simulink library "simetranss"  (R2024b)
settings: Solver=VariableStepAuto  StartTime=0.0  StopTime=10.0  RelTol=1e-3
PostLoadFcn:
  | Ts=1e-6
InitFcn:
  | Ts=1e-6
undefined symbols (not defined in the file): C, C_601, C_603, C_606, CC, Csnu, Csnubber, DiscIntNeverNeededParam, DPL, DPL1ph, FluxTable, ft2km, gcbh, h, Half, Imap2, L, L_601, L_603, L_606, Lbase, LpejoSw, Newton, R_601, R_603, R_606, Raphson, ResistanceM, Roff, Ron, RotorAngles, Rsnu, Rsnubber, Rt4, SampleTime, simetran, sps, sps_rtmsupport, StatorCurrents, T_2wind_ratio, T_Lpu, T_Lpu_pri, T_Rpu, T_Rpu_pri, T_Vpri, T_Vpri_15comp, T_Vsec, Ti, Ts_Power, Z, Zbase, Zm
libraries: fl_lib x248, ee_lib x146, nesl_utility x122, $bdroot x29, simulink x15, eeGeneralControl x2, spsStairGeneratorLib x2, artemis x1
(part 7 of 12)

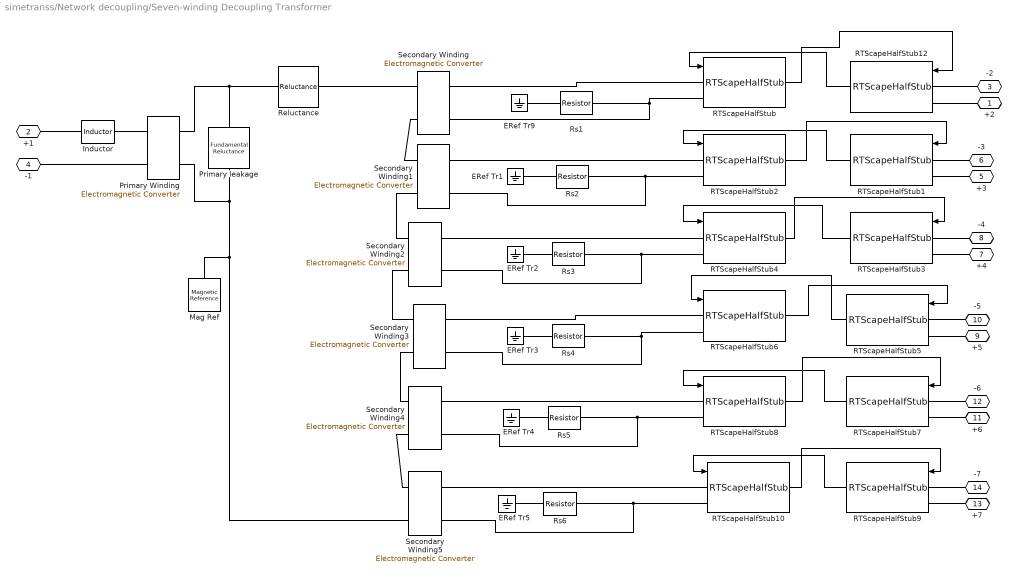
== system simetranss/Network decoupling/Seven-winding Decoupling Transformer ==
  ERef Tr{1..5,9} (6 alike) : fl_lib/Electrical/Electrical Elements/Electrical Reference
  Inductor : fl_lib/Electrical/Electrical Elements/Inductor  l=RLpri(2) H  r=RLpri(1) Ohm  g=1e-9 1/Ohm  i_specify=off  i_priority=None  i=0 A  i_nominal_specify=off  i_nominal_value=1  i_nominal_unit=A  v_specify=off  v_priority=None  v=0 V  v_nominal_specify=off  v_nominal_value=1  v_nominal_unit=V  i_L_specify=off  i_L_priority=High  i_L=0 A  i_L_nominal_specify=off  i_L_nominal_value=1  i_L_nominal_unit=A
  Mag Ref : fl_lib/Magnetic/Magnetic Elements/Magnetic Reference
      settings: InternalSimscapePortConfiguration="{\"Bottom\":[],\"Left\":[{\"id\":\"M\",\"label\":\"\",\"type\":\"foundation.magnetic.magnetic\"}],\"Right\":[],\"Top\":[]}"
  Primary Winding : fl_lib/Magnetic/Magnetic Elements/Electromagnetic Converter  Nw=Vwdn(1)  i_specify=off  i_priority=High  i=0 A  i_nominal_specify=off  i_nominal_value=1  i_nominal_unit=A  v_specify=off  v_priority=High  v=0 V  v_nominal_specify=off  v_nominal_value=1  v_nominal_unit=V  mmf_specify=off  mmf_priority=High  mmf=0 A  mmf_nominal_specify=off  mmf_nominal_value=1  mmf_nominal_unit=A  phi_specify=off  phi_priority=High  phi=0 Wb  phi_nominal_specify=off  phi_nominal_value=1  phi_nominal_unit=Wb
      settings: InternalSimscapePortConfiguration="{\"Bottom\":[],\"Left\":[{\"id\":\"p\",\"label\":\"+\",\"type\":\"foundation.electrical.electrical\"},{\"id\":\"n\",\"label\":\"-\",\"type\":\"foundation.electrical.electrical\"}],\"Right\":[{\"id\":\"N\",\"label\":\"N\",\"type\":\"foundation.magnetic.magnetic\"},{\"id\":\"S\",\"label\":\"S\",\"type\":\"foundation.magnetic.magnetic\"}],\"Top\":[]}"
  Primary leakage : fl_lib/Magnetic/Magnetic Elements/Fundamental Reluctance  R=1e8 1/H  phi_specify=off  phi_priority=None  phi=0 Wb  phi_nominal_specify=off  phi_nominal_value=1  phi_nominal_unit=Wb  mmf_specify=off  mmf_priority=None  mmf=0 A  mmf_nominal_specify=off  mmf_nominal_value=1  mmf_nominal_unit=A
      settings: InternalSimscapePortConfiguration="{\"Bottom\":[],\"Left\":[{\"id\":\"N\",\"label\":\"N\",\"type\":\"foundation.magnetic.magnetic\"}],\"Right\":[{\"id\":\"S\",\"label\":\"S\",\"type\":\"foundation.magnetic.magnetic\"}],\"Top\":[]}"
  RTScapeHalfStub : $bdroot/Network decoupling/RTScapeHalfStub  Phases=2 with differential inputs  pu=off  L=Lwdn(1)  Lpu=0.03  R=Rwdn(1)  Rpu=0.02  S_base=1e5  V_base=1000  F_base=60  Ts=Ts
  RTScapeHalfStub1 : $bdroot/Network decoupling/RTScapeHalfStub  Phases=2 with differential inputs  pu=off  L=Lwdn(2)  Lpu=0.03  R=Rwdn(2)  Rpu=0.02  S_base=1e5  V_base=1000  F_base=60  Ts=Ts
  RTScapeHalfStub10 : $bdroot/Network decoupling/RTScapeHalfStub  Phases=2 with differential inputs  pu=off  L=Lwdn(6)  Lpu=0.03  R=Rwdn(6)  Rpu=0.02  S_base=1e5  V_base=1000  F_base=60  Ts=Ts
  RTScapeHalfStub12 : $bdroot/Network decoupling/RTScapeHalfStub  Phases=2 with differential inputs  pu=off  L=Lwdn(1)  Lpu=0.03  R=Rwdn(1)  Rpu=0.02  S_base=1e5  V_base=1000  F_base=60  Ts=Ts
  RTScapeHalfStub2 : $bdroot/Network decoupling/RTScapeHalfStub  Phases=2 with differential inputs  pu=off  L=Lwdn(2)  Lpu=0.03  R=Rwdn(2)  Rpu=0.02  S_base=1e5  V_base=1000  F_base=60  Ts=Ts
  RTScapeHalfStub3 : $bdroot/Network decoupling/RTScapeHalfStub  Phases=2 with differential inputs  pu=off  L=Lwdn(3)  Lpu=0.03  R=Rwdn(3)  Rpu=0.02  S_base=1e5  V_base=1000  F_base=60  Ts=Ts
  RTScapeHalfStub4 : $bdroot/Network decoupling/RTScapeHalfStub  Phases=2 with differential inputs  pu=off  L=Lwdn(3)  Lpu=0.03  R=Rwdn(3)  Rpu=0.02  S_base=1e5  V_base=1000  F_base=60  Ts=Ts
  RTScapeHalfStub5 : $bdroot/Network decoupling/RTScapeHalfStub  Phases=2 with differential inputs  pu=off  L=Lwdn(4)  Lpu=0.03  R=Rwdn(4)  Rpu=0.02  S_base=1e5  V_base=1000  F_base=60  Ts=Ts
  RTScapeHalfStub6 : $bdroot/Network decoupling/RTScapeHalfStub  Phases=2 with differential inputs  pu=off  L=Lwdn(4)  Lpu=0.03  R=Rwdn(4)  Rpu=0.02  S_base=1e5  V_base=1000  F_base=60  Ts=Ts
  RTScapeHalfStub7 : $bdroot/Network decoupling/RTScapeHalfStub  Phases=2 with differential inputs  pu=off  L=Lwdn(5)  Lpu=0.03  R=Rwdn(5)  Rpu=0.02  S_base=1e5  V_base=1000  F_base=60  Ts=Ts
  RTScapeHalfStub8 : $bdroot/Network decoupling/RTScapeHalfStub  Phases=2 with differential inputs  pu=off  L=Lwdn(5)  Lpu=0.03  R=Rwdn(5)  Rpu=0.02  S_base=1e5  V_base=1000  F_base=60  Ts=Ts
  RTScapeHalfStub9 : $bdroot/Network decoupling/RTScapeHalfStub  Phases=2 with differential inputs  pu=off  L=Lwdn(6)  Lpu=0.03  R=Rwdn(6)  Rpu=0.02  S_base=1e5  V_base=1000  F_base=60  Ts=Ts
  Reluctance : fl_lib/Magnetic/Magnetic Elements/Reluctance  g=0.2 m  CSA=0.035*0.035 m^2  mur=8000  phi_specify=off  phi_priority=High  phi=0 Wb  phi_nominal_specify=off  phi_nominal_value=1  phi_nominal_unit=Wb  mmf_specify=off  mmf_priority=High  mmf=0 A  mmf_nominal_specify=off  mmf_nominal_value=1  mmf_nominal_unit=A
      settings: InternalSimscapePortConfiguration="{\"Bottom\":[],\"Left\":[{\"id\":\"N\",\"label\":\"N\",\"type\":\"foundation.magnetic.magnetic\"}],\"Right\":[{\"id\":\"S\",\"label\":\"S\",\"type\":\"foundation.magnetic.magnetic\"}],\"Top\":[]}"
  Rs{1..6} (6 alike) : fl_lib/Electrical/Electrical Elements/Resistor  R=Rearth Ohm  i_specify=off  i_priority=High  i=0 A  i_nominal_specify=off  i_nominal_value=1  i_nominal_unit=A  v_specify=off  v_priority=High  v=0 V  v_nominal_specify=off  v_nominal_value=1  v_nominal_unit=V
  Secondary Winding : fl_lib/Magnetic/Magnetic Elements/Electromagnetic Converter  Nw=Vwdn(1)  i_specify=off  i_priority=High  i=0 A  i_nominal_specify=off  i_nominal_value=1  i_nominal_unit=A  v_specify=off  v_priority=High  v=0 V  v_nominal_specify=off  v_nominal_value=1  v_nominal_unit=V  mmf_specify=off  mmf_priority=High  mmf=0 A  mmf_nominal_specify=off  mmf_nominal_value=1  mmf_nominal_unit=A  phi_specify=off  phi_priority=High  phi=0 Wb  phi_nominal_specify=off  phi_nominal_value=1  phi_nominal_unit=Wb
      settings: InternalSimscapePortConfiguration="{\"Bottom\":[],\"Left\":[{\"id\":\"p\",\"label\":\"+\",\"type\":\"foundation.electrical.electrical\"},{\"id\":\"n\",\"label\":\"-\",\"type\":\"foundation.electrical.electrical\"}],\"Right\":[{\"id\":\"N\",\"label\":\"N\",\"type\":\"foundation.magnetic.magnetic\"},{\"id\":\"S\",\"label\":\"S\",\"type\":\"foundation.magnetic.magnetic\"}],\"Top\":[]}"
  Secondary Winding1 : fl_lib/Magnetic/Magnetic Elements/Electromagnetic Converter  Nw=Vwdn(2)  i_specify=off  i_priority=High  i=0 A  i_nominal_specify=off  i_nominal_value=1  i_nominal_unit=A  v_specify=off  v_priority=High  v=0 V  v_nominal_specify=off  v_nominal_value=1  v_nominal_unit=V  mmf_specify=off  mmf_priority=High  mmf=0 A  mmf_nominal_specify=off  mmf_nominal_value=1  mmf_nominal_unit=A  phi_specify=off  phi_priority=High  phi=0 Wb  phi_nominal_specify=off  phi_nominal_value=1  phi_nominal_unit=Wb
      settings: InternalSimscapePortConfiguration="{\"Bottom\":[],\"Left\":[{\"id\":\"p\",\"label\":\"+\",\"type\":\"foundation.electrical.electrical\"},{\"id\":\"n\",\"label\":\"-\",\"type\":\"foundation.electrical.electrical\"}],\"Right\":[{\"id\":\"N\",\"label\":\"N\",\"type\":\"foundation.magnetic.magnetic\"},{\"id\":\"S\",\"label\":\"S\",\"type\":\"foundation.magnetic.magnetic\"}],\"Top\":[]}"
  Secondary Winding2 : fl_lib/Magnetic/Magnetic Elements/Electromagnetic Converter  Nw=Vwdn(3)  i_specify=off  i_priority=High  i=0 A  i_nominal_specify=off  i_nominal_value=1  i_nominal_unit=A  v_specify=off  v_priority=High  v=0 V  v_nominal_specify=off  v_nominal_value=1  v_nominal_unit=V  mmf_specify=off  mmf_priority=High  mmf=0 A  mmf_nominal_specify=off  mmf_nominal_value=1  mmf_nominal_unit=A  phi_specify=off  phi_priority=High  phi=0 Wb  phi_nominal_specify=off  phi_nominal_value=1  phi_nominal_unit=Wb
      settings: InternalSimscapePortConfiguration="{\"Bottom\":[],\"Left\":[{\"id\":\"p\",\"label\":\"+\",\"type\":\"foundation.electrical.electrical\"},{\"id\":\"n\",\"label\":\"-\",\"type\":\"foundation.electrical.electrical\"}],\"Right\":[{\"id\":\"N\",\"label\":\"N\",\"type\":\"foundation.magnetic.magnetic\"},{\"id\":\"S\",\"label\":\"S\",\"type\":\"foundation.magnetic.magnetic\"}],\"Top\":[]}"
  Secondary Winding3 : fl_lib/Magnetic/Magnetic Elements/Electromagnetic Converter  Nw=Vwdn(4)  i_specify=off  i_priority=High  i=0 A  i_nominal_specify=off  i_nominal_value=1  i_nominal_unit=A  v_specify=off  v_priority=High  v=0 V  v_nominal_specify=off  v_nominal_value=1  v_nominal_unit=V  mmf_specify=off  mmf_priority=High  mmf=0 A  mmf_nominal_specify=off  mmf_nominal_value=1  mmf_nominal_unit=A  phi_specify=off  phi_priority=High  phi=0 Wb  phi_nominal_specify=off  phi_nominal_value=1  phi_nominal_unit=Wb
      settings: InternalSimscapePortConfiguration="{\"Bottom\":[],\"Left\":[{\"id\":\"p\",\"label\":\"+\",\"type\":\"foundation.electrical.electrical\"},{\"id\":\"n\",\"label\":\"-\",\"type\":\"foundation.electrical.electrical\"}],\"Right\":[{\"id\":\"N\",\"label\":\"N\",\"type\":\"foundation.magnetic.magnetic\"},{\"id\":\"S\",\"label\":\"S\",\"type\":\"foundation.magnetic.magnetic\"}],\"Top\":[]}"
  Secondary Winding4 : fl_lib/Magnetic/Magnetic Elements/Electromagnetic Converter  Nw=Vwdn(5)  i_specify=off  i_priority=High  i=0 A  i_nominal_specify=off  i_nominal_value=1  i_nominal_unit=A  v_specify=off  v_priority=High  v=0 V  v_nominal_specify=off  v_nominal_value=1  v_nominal_unit=V  mmf_specify=off  mmf_priority=High  mmf=0 A  mmf_nominal_specify=off  mmf_nominal_value=1  mmf_nominal_unit=A  phi_specify=off  phi_priority=High  phi=0 Wb  phi_nominal_specify=off  phi_nominal_value=1  phi_nominal_unit=Wb
      settings: InternalSimscapePortConfiguration="{\"Bottom\":[],\"Left\":[{\"id\":\"p\",\"label\":\"+\",\"type\":\"foundation.electrical.electrical\"},{\"id\":\"n\",\"label\":\"-\",\"type\":\"foundation.electrical.electrical\"}],\"Right\":[{\"id\":\"N\",\"label\":\"N\",\"type\":\"foundation.magnetic.magnetic\"},{\"id\":\"S\",\"label\":\"S\",\"type\":\"foundation.magnetic.magnetic\"}],\"Top\":[]}"
  Secondary Winding5 : fl_lib/Magnetic/Magnetic Elements/Electromagnetic Converter  Nw=Vwdn(6)  i_specify=off  i_priority=High  i=0 A  i_nominal_specify=off  i_nominal_value=1  i_nominal_unit=A  v_specify=off  v_priority=High  v=0 V  v_nominal_specify=off  v_nominal_value=1  v_nominal_unit=V  mmf_specify=off  mmf_priority=High  mmf=0 A  mmf_nominal_specify=off  mmf_nominal_value=1  mmf_nominal_unit=A  phi_specify=off  phi_priority=High  phi=0 Wb  phi_nominal_specify=off  phi_nominal_value=1  phi_nominal_unit=Wb
      settings: InternalSimscapePortConfiguration="{\"Bottom\":[],\"Left\":[{\"id\":\"p\",\"label\":\"+\",\"type\":\"foundation.electrical.electrical\"},{\"id\":\"n\",\"label\":\"-\",\"type\":\"foundation.electrical.electrical\"}],\"Right\":[{\"id\":\"N\",\"label\":\"N\",\"type\":\"foundation.magnetic.magnetic\"},{\"id\":\"S\",\"label\":\"S\",\"type\":\"foundation.magnetic.magnetic\"}],\"Top\":[]}"
  +2 : PMIOPort  Side=Right
  +1 : PMIOPort  Port=2  Side=Left
  -2 : PMIOPort  Port=3  Side=Right
  -1 : PMIOPort  Port=4  Side=Left
  +3 : PMIOPort  Port=5  Side=Right
  -3 : PMIOPort  Port=6  Side=Right
  +4 : PMIOPort  Port=7  Side=Right
  -4 : PMIOPort  Port=8  Side=Right
  +5 : PMIOPort  Port=9  Side=Right
  -5 : PMIOPort  Port=10  Side=Right
  +6 : PMIOPort  Port=11  Side=Right
  -6 : PMIOPort  Port=12  Side=Right
  +7 : PMIOPort  Port=13  Side=Right
  -7 : PMIOPort  Port=14  Side=Right
  wires:
  RTScapeHalfStub/1 -> RTScapeHalfStub12/1
  RTScapeHalfStub12/1 -> RTScapeHalfStub/1
  RTScapeHalfStub1/1 -> RTScapeHalfStub2/1
  RTScapeHalfStub2/1 -> RTScapeHalfStub1/1
  RTScapeHalfStub4/1 -> RTScapeHalfStub3/1
  RTScapeHalfStub3/1 -> RTScapeHalfStub4/1
  RTScapeHalfStub5/1 -> RTScapeHalfStub6/1
  RTScapeHalfStub6/1 -> RTScapeHalfStub5/1
  RTScapeHalfStub8/1 -> RTScapeHalfStub7/1
  RTScapeHalfStub7/1 -> RTScapeHalfStub8/1
  RTScapeHalfStub9/1 -> RTScapeHalfStub10/1
  RTScapeHalfStub10/1 -> RTScapeHalfStub9/1
  connections:
  Secondary Winding4/RConn1 -- Secondary Winding5/RConn2
  Secondary Winding3/RConn1 -- Secondary Winding4/RConn2
  Secondary Winding2/RConn1 -- Secondary Winding3/RConn2
  Secondary Winding1/RConn1 -- Secondary Winding2/RConn2
  Secondary Winding1/RConn2 -- Secondary Winding/RConn1
  Reluctance/RConn1 -- Secondary Winding/RConn2
  Primary leakage/RConn1 -- Primary Winding/RConn2 -- Mag Ref/LConn1 -- Secondary Winding5/RConn1
  Primary leakage/LConn1 -- Reluctance/LConn1 -- Primary Winding/RConn1
  -1/RConn1 -- Primary Winding/LConn2
  Inductor/RConn1 -- Primary Winding/LConn1
  Secondary Winding/LConn1 -- RTScapeHalfStub/LConn2 -- Rs1/RConn1
  Rs1/LConn1 -- ERef Tr9/LConn1
  RTScapeHalfStub12/LConn2 -- +2/RConn1
  RTScapeHalfStub12/LConn1 -- -2/RConn1
  RTScapeHalfStub/LConn1 -- Secondary Winding/LConn2
  Rs2/RConn1 -- RTScapeHalfStub2/LConn2 -- Secondary Winding1/LConn1
  RTScapeHalfStub2/LConn1 -- Secondary Winding1/LConn2
  RTScapeHalfStub1/LConn2 -- +3/RConn1
  RTScapeHalfStub1/LConn1 -- -3/RConn1
  Rs2/LConn1 -- ERef Tr1/LConn1
  Rs3/RConn1 -- RTScapeHalfStub4/LConn2 -- Secondary Winding2/LConn1
  ERef Tr2/LConn1 -- Rs3/LConn1
  RTScapeHalfStub4/LConn1 -- Secondary Winding2/LConn2
  RTScapeHalfStub3/LConn1 -- -4/RConn1
  RTScapeHalfStub3/LConn2 -- +4/RConn1
  Rs4/RConn1 -- RTScapeHalfStub6/LConn2 -- Secondary Winding3/LConn1
  RTScapeHalfStub5/LConn1 -- -5/RConn1
  RTScapeHalfStub6/LConn1 -- Secondary Winding3/LConn2
  ERef Tr3/LConn1 -- Rs4/LConn1
  RTScapeHalfStub5/LConn2 -- +5/RConn1
  Rs5/RConn1 -- RTScapeHalfStub8/LConn2 -- Secondary Winding4/LConn1
  RTScapeHalfStub7/LConn2 -- +6/RConn1
  ERef Tr4/LConn1 -- Rs5/LConn1
  RTScapeHalfStub7/LConn1 -- -6/RConn1
  RTScapeHalfStub8/LConn1 -- Secondary Winding4/LConn2
  Rs6/RConn1 -- RTScapeHalfStub10/LConn2 -- Secondary Winding5/LConn1
  RTScapeHalfStub10/LConn1 -- Secondary Winding5/LConn2
  ERef Tr5/LConn1 -- Rs6/LConn1
  RTScapeHalfStub9/LConn1 -- -7/RConn1
  RTScapeHalfStub9/LConn2 -- +7/RConn1
  +1/RConn1 -- Inductor/LConn1

== system simetranss/Network decoupling/Three-Phase 2-Windings Decoupling Transformer ==
  Signal Specification : SignalSpecification  Dimensions=3
  Signal Specification1 : SignalSpecification  Dimensions=3
  Switch : Switch  Criteria=u2 > Threshold  Threshold=0.5  SaturateOnIntegerOverflow=off  InputSameDT=off
  Switch1 : Switch  Criteria=u2 > Threshold  Threshold=0.5  SaturateOnIntegerOverflow=off  InputSameDT=off
  Terminator : Terminator
  Terminator1 : Terminator
  del{1..4} (4 alike) : UnitDelay  SampleTime=Ts  HasFrameUpgradeWarning=on
  hinpri : Ground
  hinsec : Ground
  houtpri : Terminator
  houtsec : Terminator
  path : Constant
  pri : Subsystem
  sec : Subsystem
  ABC : PMIOPort  Side=Left
  N : PMIOPort  Port=2  Side=Left
  abc : PMIOPort  Port=3  Side=Right
  n : PMIOPort  Port=4  Side=Right
  wires:
  pri/1(Out1) -> Signal Specification1/1, Terminator/1, houtpri/1
  sec/1(Out1) -> Terminator1/1, houtsec/1, Signal Specification/1
  Switch/1 -> pri/1(In1)
  del1/1 -> Switch/3
  hinpri/1 -> del4/1
  path/1 -> Switch/2, Switch1/2
  del2/1 -> Switch1/3
  Switch1/1 -> sec/1(In1)
  hinsec/1 -> del3/1
  Signal Specification/1 -> del1/1
  Signal Specification1/1 -> del2/1
  del3/1 -> Switch1/1
  del4/1 -> Switch/1
  connections:
  ABC/RConn1 -- pri/LConn1
  N/RConn1 -- pri/LConn2
  abc/RConn1 -- sec/RConn1
  n/RConn1 -- sec/RConn2

== system simetranss/Passive/MATE Single-Phase Load ==
  C : Subsystem  Commented=on
  RLseries : Subsystem
  a : PMIOPort  Side=Left
  connections:
  C/LConn1 -- a/RConn1 -- RLseries/LConn1

== system simetranss/Passive/MATE Unbalanced Load ==
  C : Subsystem  Commented=on
  RLseries : Subsystem
  abc : PMIOPort  Side=Left
  connections:
  abc/RConn1 -- C/LConn1 -- RLseries/LConn1

== system simetranss/Passive/MATE Unbalanced LoadDEV1 ==
  C : Subsystem  Commented=on
  CD : Subsystem  Commented=on
  RLseries : Subsystem
  RLseriesD : Subsystem
  abc : PMIOPort  Side=Left
  connections:
  abc/RConn1 -- RLseriesD/LConn1 -- RLseries/LConn1 -- CD/LConn1 -- C/LConn1

== system simetranss/Passive/RLC ==
  note: RLC parallel LC parallel
  note: RLC series LC series
  note: L RLseries RLparallel
  note: C RCseries RCparallel
  C : ee_lib/Passive/Capacitor  Commented=on  cap_option=ee.enum.passive.capacitor.capOption.const  c=Capacitance F  Cvec=[1e-05, 1e-06] F  Vvec=[0, 10] V  CV_table_symmetry=ee.enum.passive.capacitor.tableSymmetry.yes  f_vec=[1, 10] kHz  DFext_vec=[.8, 1.2]  enable_C_tol=ee.enum.toleranceApplication.none  averaging_period=0 s  C_tol=5  tol_distribution=ee.enum.toleranceDistribution.uniform  nSigma=4  r=Resistance2 Ohm  g=0 1/Ohm  enable_operating_limits=ee.enum.enable.no  operating_limit_action=ee.enum.passive.reportOpLim.warn  max_working_voltage_range=[-25, 25] V  power_rating=1 W  maxTemperature=85 degC  thermalEnable=false  thermalMass=1 J/K  fault_action=simscape.enum.assert.action.none  t_fault=1 s  i_specify=off  i_priority=None  i=0 A  i_nominal_specify=off  i_nominal_value=1  i_nominal_unit=A  v_specify=off  v_priority=None  v=0 V  v_nominal_specify=off  v_nominal_value=1  v_nominal_unit=V  vc_specify=off  vc_priority=High  vc=0 V  vc_nominal_specify=off  vc_nominal_value=1  vc_nominal_unit=V  T_specify=off  T_priority=None  T=298.15 K  T_nominal_specify=off  T_nominal_value=1  T_nominal_unit=K
  L : ee_lib/Passive/Inductor  l=Inductance H  enable_L_tol=ee.enum.toleranceApplication.none  L_tol=20  tol_distribution=ee.enum.toleranceDistribution.uniform  nSigma=4  r=Resistance2 Ohm  g=0 1/Ohm  enable_operating_limits=ee.enum.enable.no  operating_limit_action=ee.enum.passive.reportOpLim.warn  max_working_current=1 A  power_rating=1 W  fault_action=simscape.enum.assert.action.none  t_fault=1 s  i_L_specify=off  i_L_priority=High  i_L=0 A  i_L_nominal_specify=off  i_L_nominal_value=1  i_L_nominal_unit=A
  R : ee_lib/Passive/Resistor  R=Resistance Ohm  enable_R_tol=ee.enum.toleranceApplication.none  R_tol=5  tol_distribution=ee.enum.toleranceDistribution.uniform  nSigma=4  enable_operating_limits=ee.enum.enable.no  operating_limit_action=ee.enum.passive.reportOpLim.warn  power_rating=1 W  max_working_voltage=100 V  noise_mode=ee.enum.sources.noise.Disabled  Tdevice=25 degC  sample_time=1e-3 s  repeatability=ee.enum.ic.repeatability.notRepeatable  user_seed=0  auto_seed=3102854422  fault_action=simscape.enum.assert.action.none  t_fault=1 s  power_derating_T1=70 degC  power_derating_T2=155 degC  operating_temperature_range_vec=[-50, 150] degC  alpha=3.93e-3 1/K  Tmeas=25 degC  thermal_mass=100 J/K  temperature_specify=off  temperature_priority=High  temperature=298.15 K  temperature_nominal_specify=off  temperature_nominal_value=1  temperature_nominal_unit=K
  RLCp_1 : ee_lib/Passive/Capacitor  Commented=on  cap_option=ee.enum.passive.capacitor.capOption.const  c=Capacitance F  Cvec=[1e-05, 1e-06] F  Vvec=[0, 10] V  CV_table_symmetry=ee.enum.passive.capacitor.tableSymmetry.yes  f_vec=[1, 10] kHz  DFext_vec=[.8, 1.2]  enable_C_tol=ee.enum.toleranceApplication.none  averaging_period=0 s  C_tol=5  tol_distribution=ee.enum.toleranceDistribution.uniform  nSigma=4  r=0 Ohm  g=1/Resistance2 1/Ohm  enable_operating_limits=ee.enum.enable.no  operating_limit_action=ee.enum.passive.reportOpLim.warn  max_working_voltage_range=[-25, 25] V  power_rating=1 W  maxTemperature=85 degC  thermalEnable=false  thermalMass=1 J/K  fault_action=simscape.enum.assert.action.none  t_fault=1 s  i_specify=off  i_priority=None  i=0 A  i_nominal_specify=off  i_nominal_value=1  i_nominal_unit=A  v_specify=off  v_priority=None  v=0 V  v_nominal_specify=off  v_nominal_value=1  v_nominal_unit=V  vc_specify=off  vc_priority=High  vc=0 V  vc_nominal_specify=off  vc_nominal_value=1  vc_nominal_unit=V  T_specify=off  T_priority=None  T=298.15 K  T_nominal_specify=off  T_nominal_value=1  T_nominal_unit=K
  RLCp_2 : ee_lib/Passive/Inductor  Commented=on  l=Inductance H  enable_L_tol=ee.enum.toleranceApplication.none  L_tol=20  tol_distribution=ee.enum.toleranceDistribution.uniform  nSigma=4  r=0 Ohm  g=0 1/Ohm  enable_operating_limits=ee.enum.enable.no  operating_limit_action=ee.enum.passive.reportOpLim.warn  max_working_current=1 A  power_rating=1 W  fault_action=simscape.enum.assert.action.none  t_fault=1 s  i_L_specify=off  i_L_priority=High  i_L=0 A  i_L_nominal_specify=off  i_L_nominal_value=1  i_L_nominal_unit=A
  RLCs_1 : ee_lib/Passive/Capacitor  Commented=on  cap_option=ee.enum.passive.capacitor.capOption.const  c=Capacitance F  Cvec=[1e-05, 1e-06] F  Vvec=[0, 10] V  CV_table_symmetry=ee.enum.passive.capacitor.tableSymmetry.yes  f_vec=[1, 10] kHz  DFext_vec=[.8, 1.2]  enable_C_tol=ee.enum.toleranceApplication.none  averaging_period=0 s  C_tol=5  tol_distribution=ee.enum.toleranceDistribution.uniform  nSigma=4  r=0 Ohm  g=0 1/Ohm  enable_operating_limits=ee.enum.enable.no  operating_limit_action=ee.enum.passive.reportOpLim.warn  max_working_voltage_range=[-25, 25] V  power_rating=1 W  maxTemperature=85 degC  thermalEnable=false  thermalMass=1 J/K  fault_action=simscape.enum.assert.action.none  t_fault=1 s  i_specify=off  i_priority=None  i=0 A  i_nominal_specify=off  i_nominal_value=1  i_nominal_unit=A  v_specify=off  v_priority=None  v=0 V  v_nominal_specify=off  v_nominal_value=1  v_nominal_unit=V  vc_specify=off  vc_priority=High  vc=0 V  vc_nominal_specify=off  vc_nominal_value=1  vc_nominal_unit=V  T_specify=off  T_priority=None  T=298.15 K  T_nominal_specify=off  T_nominal_value=1  T_nominal_unit=K
  RLCs_2 : ee_lib/Passive/Inductor  Commented=on  l=Inductance H  enable_L_tol=ee.enum.toleranceApplication.none  L_tol=20  tol_distribution=ee.enum.toleranceDistribution.uniform  nSigma=4  r=Resistance2 Ohm  g=0 1/Ohm  enable_operating_limits=ee.enum.enable.no  operating_limit_action=ee.enum.passive.reportOpLim.warn  max_working_current=1 A  power_rating=1 W  fault_action=simscape.enum.assert.action.none  t_fault=1 s  i_L_specify=off  i_L_priority=High  i_L=0 A  i_L_nominal_specify=off  i_L_nominal_value=1  i_L_nominal_unit=A
  + : PMIOPort  Side=Left
  - : PMIOPort  Port=2  Side=Right
  connections:
  C/LConn1 -- +/RConn1 -- R/RConn1 -- L/LConn1 -- RLCs_1/LConn1 -- RLCp_2/LConn1 -- RLCp_1/LConn1
  RLCs_2/LConn1 -- RLCs_1/RConn1
  L/RConn1 -- -/RConn1 -- R/LConn1 -- C/RConn1 -- RLCs_2/RConn1 -- RLCp_2/RConn1 -- RLCp_1/RConn1

== system simetranss/Passive/RLC(3ph) ==
  RLC3 : ee_lib/Passive/RLC Assemblies/RLC (Three-Phase)  port_option=ee.enum.threePhasePort.composite  component_structure=ee.enum.rlc.structure.SeriesRLC  R=Resistance Ohm  L=Inductance H  C=Capacitance F  R_parasitic=0 Ohm  G_parasitic=0 1/Ohm  IL_specify=off  IL_priority=High  IL=[0, 0, 0] A  IL_nominal_specify=off  IL_nominal_value=1  IL_nominal_unit=A  VC_specify=off  VC_priority=High  VC=[0, 0, 0] V  VC_nominal_specify=off  VC_nominal_value=1  VC_nominal_unit=V
      settings: InternalSimscapePortConfiguration="{\"Bottom\":[],\"Left\":[{\"id\":\"N1\",\"label\":\"~1\",\"type\":\"foundation.electrical.three_phase\"}],\"Right\":[{\"id\":\"N2\",\"label\":\"~2\",\"type\":\"foundation.electrical.three_phase\"}],\"Top\":[]}"
  + : PMIOPort  Side=Left
  - : PMIOPort  Port=2  Side=Right
  connections:
  RLC3/RConn1 -- -/RConn1
  RLC3/LConn1 -- +/RConn1

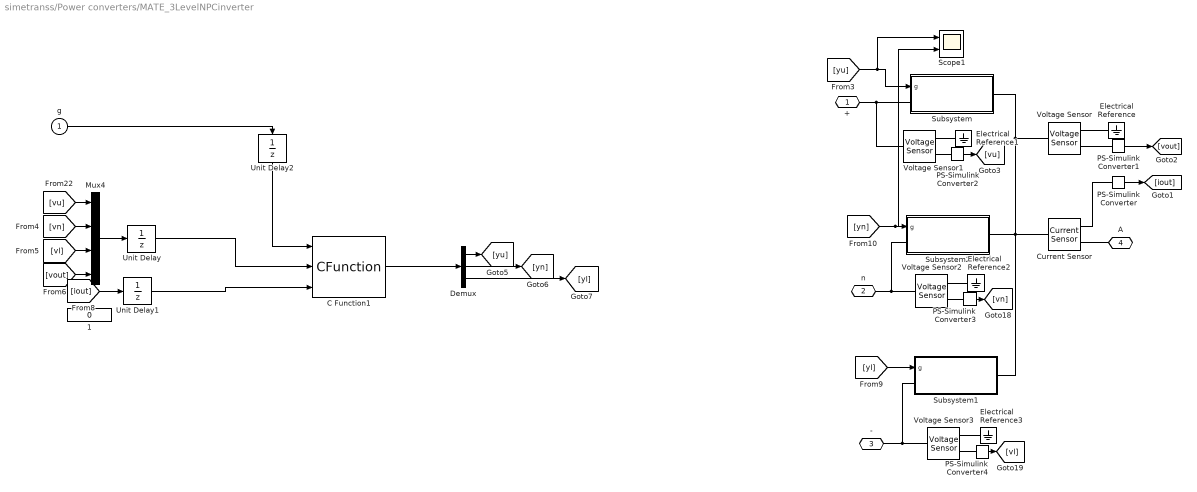
== system simetranss/Power converters/MATE_3LevelNPCinverter ==
  g : Inport
  1 : Constant  Value=0
  C Function1 : CFunction  OutputCode=|  InitializeConditionsCode=status_old=0;  CodegenOutputCode=|  CodegenInitializeConditionsCode=status_old=0;  CustomCodeSettingLocation=ModelConfigurationParameters
      OutputCode=|
      | {
      |     double status;
      | 
      |     //InputRealPtrsType gg      = ssGetInputPortRealSignalPtrs(S,0);
      |     //InputRealPtrsType Vtermm  = ssGetInputPortRealSignalPtrs(S,1);
      |     //InputRealPtrsType ioutt   = ssGetInputPortRealSignalPtrs(S,2);
      |     //InputRealPtrsType tol     = ssGetInputPortRealSignalPtrs(S,3);
      | 
      | 
      |     //real_T            *sw       =  ssGetOutputPortRealSignal(S,0);  // sw
      |     //real_T			  *stat     =  ssGetOutputPortRealSignal(S,1);  // status
      | 
      | 
      | 
      |     //mexPrintf("OUTPUTpause:\n");
      |     //mexEvalString("pause(2);");
      | 
      | 
      | 
      |     //real_T *status_old    = (real_T*) ssGetDWork(S,0);
      |     //real_T status[1];
      | 
      | 
      |     //real_T  g[4];
      |     //real_T  Vterm[4];
      |  
      | 
      |     //real_T iout[1];
      | 
      |    // *(g+0)= *gg[0];
      |    // *(g+1)= *gg[1];
      |    // *(g+2)= *gg[2];
      |    // *(g+3)= *gg[3];
      | 
      |    // *(Vterm+0)= *Vtermm[0];
      |    // *(Vterm+1)= *Vtermm[1];
      |    // *(Vterm+2)= *Vtermm[2];
      |    // *(Vterm+3)= *Vtermm[3];
      | 
      |    // iout= *ioutt[0];
      | 
      | 
      |  
      | 
      | 
      |     if (*(g+0)>0.5 && *(g+1)>0.5) {
      |         *(sw+0)=1;*(sw+1)=0;*(sw+2)=0;status=1;
      |     }
      |     else if (*(g+2)>0.5  && *(g+3)>0.5) {
      |         *(sw+0)=0;*(sw+1)=0;*(sw+2)=1;status=2;
      |     }
      |     else if (*(g+1)>0.5  && *(g+2)>0.5) {
      |         *(sw+0)=0;*(sw+1)=1;*(sw+2)=0;status=3;
      |     }
      |     else if (*(g+1)>0.5 && iout>0) {
      |         *(sw+0)=0;*(sw+1)=1;*(sw+2)=0;status=4;
      |     }
      |     else if (*(g+2)>0.5 && iout<0) {
      |         *(sw+0)=0;*(sw+1)=1;*(sw+2)=0;status=5;
      |     }
      |     else if ( (iout>0 && status_old<=6)) { //|| (*(iout>tol[0] && status_old>5) )  {
      |         *(sw+0)=0;*(sw+1)=0;*(sw+2)=1;status=6;
      |     }
      |     else if ( (iout<0 && status_old<=5) || (iout<0 && status_old==7) ) { // || (iout<(0-tol[0]) && status_old[0]>5)   ) {
      |         *(sw+0)=1;*(sw+1)=0;*(sw+2)=0;status=7;
      |     }
      |     else if ( (*(Vterm+3)>*(Vterm+1) && *(g+2)>0.5) || (*(Vterm+3)<*(Vterm+1)  && *(g+1)>0.5) ) {
      |         *(sw+0)=0;*(sw+1)=1;*(sw+2)=0;status=8;
      |     }
      |     else if (*(Vterm+3)>*(Vterm+0)) {
      |         *(sw+0)=1;*(sw+1)=0;*(sw+2)=0;status=9;
      |     }
      |     else if (*(Vterm+3)<*(Vterm+2)) {
      |         *(sw+0)=0;*(sw+1)=0;*(sw+2)=1;status=10;
      |     }
      |     else {
      |         *(sw+0)=0;*(sw+1)=0;*(sw+2)=0;status=11;
      |     }
      | 
      | 
      | 
      |     status_old=status;
      | 
      | 
      | }
      CodegenOutputCode=|
      | {
      |     double status;
      | 
      |     //InputRealPtrsType gg      = ssGetInputPortRealSignalPtrs(S,0);
      |     //InputRealPtrsType Vtermm  = ssGetInputPortRealSignalPtrs(S,1);
      |     //InputRealPtrsType ioutt   = ssGetInputPortRealSignalPtrs(S,2);
      |     //InputRealPtrsType tol     = ssGetInputPortRealSignalPtrs(S,3);
      | 
      | 
      |     //real_T            *sw       =  ssGetOutputPortRealSignal(S,0);  // sw
      |     //real_T			  *stat     =  ssGetOutputPortRealSignal(S,1);  // status
      | 
      | 
      | 
      |     //mexPrintf("OUTPUTpause:\n");
      |     //mexEvalString("pause(2);");
      | 
      | 
      | 
      |     //real_T *status_old    = (real_T*) ssGetDWork(S,0);
      |     //real_T status[1];
      | 
      | 
      |     //real_T  g[4];
      |     //real_T  Vterm[4];
      |  
      | 
      |     //real_T iout[1];
      | 
      |    // *(g+0)= *gg[0];
      |    // *(g+1)= *gg[1];
      |    // *(g+2)= *gg[2];
      |    // *(g+3)= *gg[3];
      | 
      |    // *(Vterm+0)= *Vtermm[0];
      |    // *(Vterm+1)= *Vtermm[1];
      |    // *(Vterm+2)= *Vtermm[2];
      |    // *(Vterm+3)= *Vtermm[3];
      | 
      |    // iout= *ioutt[0];
      | 
      | 
      |  
      | 
      | 
      |     if (*(g+0)>0.5 && *(g+1)>0.5) {
      |         *(sw+0)=1;*(sw+1)=0;*(sw+2)=0;status=1;
      |     }
      |     else if (*(g+2)>0.5  && *(g+3)>0.5) {
      |         *(sw+0)=0;*(sw+1)=0;*(sw+2)=1;status=2;
      |     }
      |     else if (*(g+1)>0.5  && *(g+2)>0.5) {
      |         *(sw+0)=0;*(sw+1)=1;*(sw+2)=0;status=3;
      |     }
      |     else if (*(g+1)>0.5 && iout>0) {
      |         *(sw+0)=0;*(sw+1)=1;*(sw+2)=0;status=4;
      |     }
      |     else if (*(g+2)>0.5 && iout<0) {
      |         *(sw+0)=0;*(sw+1)=1;*(sw+2)=0;status=5;
      |     }
      |     else if ( (iout>0 && status_old<=6)) { //|| (*(iout>tol[0] && status_old>5) )  {
      |         *(sw+0)=0;*(sw+1)=0;*(sw+2)=1;status=6;
      |     }
      |     else if ( (iout<0 && status_old<=5) || (iout<0 && status_old==7) ) { // || (iout<(0-tol[0]) && status_old[0]>5)   ) {
      |         *(sw+0)=1;*(sw+1)=0;*(sw+2)=0;status=7;
      |     }
      |     else if ( (*(Vterm+3)>*(Vterm+1) && *(g+2)>0.5) || (*(Vterm+3)<*(Vterm+1)  && *(g+1)>0.5) ) {
      |         *(sw+0)=0;*(sw+1)=1;*(sw+2)=0;status=8;
      |     }
      |     else if (*(Vterm+3)>*(Vterm+0)) {
      |         *(sw+0)=1;*(sw+1)=0;*(sw+2)=0;status=9;
      |     }
      |     else if (*(Vterm+3)<*(Vterm+2)) {
      |         *(sw+0)=0;*(sw+1)=0;*(sw+2)=1;status=10;
      |     }
      |     else {
      |         *(sw+0)=0;*(sw+1)=0;*(sw+2)=0;status=11;
      |     }
      | 
      | 
      | 
      |     status_old=status;
      | 
      | 
      | }
  Current Sensor : fl_lib/Electrical/Electrical Sensors/Current Sensor
  Demux : Demux  Outputs=3
  Electrical Reference{,1..3} (4 alike) : fl_lib/Electrical/Electrical Elements/Electrical Reference
  Mux4 : Mux
  PS-Simulink Converter{,1..4} (5 alike) : nesl_utility/PS-Simulink Converter  PhysicalDomain=network_engine_domain  SubClassName=ps_output  LeftPortType=input  RightPortType=output  PseudoPeriodic=off  Frequencies=[]  VectorFormat=inherit  Unit=inherit  AffineConversion=off
  Scope1 : Scope  NumInputPorts=2
  Subsystem : Subsystem
  Subsystem1 : Subsystem
  Subsystem2 : Subsystem
  Unit Delay : UnitDelay  SampleTime=Ts  HasFrameUpgradeWarning=on
  Unit Delay1 : UnitDelay  SampleTime=Ts  HasFrameUpgradeWarning=on
  Unit Delay2 : UnitDelay  SampleTime=Ts  HasFrameUpgradeWarning=on
  Voltage Sensor{,1..3} (4 alike) : fl_lib/Electrical/Electrical Sensors/Voltage Sensor
  + : PMIOPort  Side=Left
  n : PMIOPort  Port=2  Side=Left
  - : PMIOPort  Port=3  Side=Left
  A : PMIOPort  Port=4  Side=Right
  wires:
  Mux4/1 -> Unit Delay/1
  Demux/2 -> [yn]
  [vu] -> Mux4/1
  [vn] -> Mux4/2
  [vl] -> Mux4/3
  [vout] -> Mux4/4
  g/1 -> Unit Delay2/1
  Demux/3 -> [yl]
  Demux/1 -> [yu]
  [yu] -> Scope1/1, Subsystem/1(g)
  [yl] -> Subsystem1/1(g)
  [yn] -> Subsystem2/1(g), Scope1/2
  PS-Simulink Converter/1 -> [iout]
  PS-Simulink Converter1/1 -> [vout]
  PS-Simulink Converter2/1 -> [vu]
  PS-Simulink Converter3/1 -> [vn]
  PS-Simulink Converter4/1 -> [vl]
  [iout] -> Unit Delay1/1
  C Function1/1 -> Demux/1
  Unit Delay/1 -> C Function1/2
  Unit Delay1/1 -> C Function1/3
  Unit Delay2/1 -> C Function1/1
  connections:
  +/RConn1 -- Subsystem/LConn1 -- Voltage Sensor1/LConn1
  -/RConn1 -- Subsystem1/LConn1 -- Voltage Sensor3/LConn1
  Current Sensor/LConn1 -- Subsystem1/RConn1 -- Subsystem2/RConn1 -- Subsystem/RConn1 -- Voltage Sensor/LConn1
  n/RConn1 -- Subsystem2/LConn1 -- Voltage Sensor2/LConn1
  A/RConn1 -- Current Sensor/RConn2
  PS-Simulink Converter/LConn1 -- Current Sensor/RConn1
  Voltage Sensor/RConn2 -- Electrical Reference/LConn1
  Voltage Sensor/RConn1 -- PS-Simulink Converter1/LConn1
  Voltage Sensor1/RConn2 -- Electrical Reference1/LConn1
  Voltage Sensor1/RConn1 -- PS-Simulink Converter2/LConn1
  Voltage Sensor2/RConn1 -- PS-Simulink Converter3/LConn1
  Voltage Sensor2/RConn2 -- Electrical Reference2/LConn1
  Voltage Sensor3/RConn2 -- Electrical Reference3/LConn1
  Voltage Sensor3/RConn1 -- PS-Simulink Converter4/LConn1

== system simetranss/Power converters/MATE_3LevelNPCinverter(3ph) ==
  gate : Inport
  Demux1 : Demux  Outputs=[4 4 4]
  MATE_3LevelNPCinverter : $bdroot/Power converters/MATE_3LevelNPCinverter  Arms=1  SnubberResistance=Rsnu  SnubberCapacitance=Csnu  Device=IGBT / Diodes  Ron=1e-3  Vf=1  ihiz=999
  MATE_3LevelNPCinverter1 : $bdroot/Power converters/MATE_3LevelNPCinverter  Arms=1  SnubberResistance=Rsnu  SnubberCapacitance=Csnu  Device=IGBT / Diodes  Ron=1e-3  Vf=1  ihiz=999
  MATE_3LevelNPCinverter2 : $bdroot/Power converters/MATE_3LevelNPCinverter  Arms=1  SnubberResistance=Rsnu  SnubberCapacitance=Csnu  Device=IGBT / Diodes  Ron=1e-3  Vf=1  ihiz=999
  Phase Splitter2 : ee_lib/Connectors & References/Phase Splitter
  + : PMIOPort  Side=Left
  n : PMIOPort  Port=2  Side=Left
  ABC : PMIOPort  Port=3  Side=Right
  - : PMIOPort  Port=4  Side=Left
  wires:
  gate/1 -> Demux1/1
  Demux1/1 -> MATE_3LevelNPCinverter/1
  Demux1/2 -> MATE_3LevelNPCinverter1/1
  Demux1/3 -> MATE_3LevelNPCinverter2/1
  connections:
  +/RConn1 -- MATE_3LevelNPCinverter/LConn1 -- MATE_3LevelNPCinverter2/LConn1 -- MATE_3LevelNPCinverter1/LConn1
  n/RConn1 -- MATE_3LevelNPCinverter2/LConn2 -- MATE_3LevelNPCinverter1/LConn2 -- MATE_3LevelNPCinverter/LConn2
  -/RConn1 -- MATE_3LevelNPCinverter2/LConn3 -- MATE_3LevelNPCinverter1/LConn3 -- MATE_3LevelNPCinverter/LConn3
  Phase Splitter2/LConn1 -- ABC/RConn1
  MATE_3LevelNPCinverter1/RConn1 -- Phase Splitter2/RConn2
  MATE_3LevelNPCinverter/RConn1 -- Phase Splitter2/RConn1
  MATE_3LevelNPCinverter2/RConn1 -- Phase Splitter2/RConn3

== system simetranss/Power converters/MATE_Cascaded_Hbridge_Inverter ==
  note: note i is current going out from + terminal
  g : Inport
  Vdc : Inport  Port=2
  Bus Creator : BusCreator  Inputs=2
  Controlled Current Source : fl_lib/Electrical/Electrical Sources/Controlled Current Source
  Divide : Product  Inputs=/
  PS-Simulink Converter2 : nesl_utility/PS-Simulink Converter  PhysicalDomain=network_engine_domain  SubClassName=ps_output  LeftPortType=input  RightPortType=output  PseudoPeriodic=off  Frequencies=[]  VectorFormat=inherit  Unit=inherit  AffineConversion=off
  S-Function : S-Function  FunctionName=MateHBridgeInverter  Parameters=nbc,Ts,ron,roff  SFunctionDeploymentMode=off  EnableBusSupport=off
  Saturation : Saturate  UpperLimit=1e9  LowerLimit=1e-9
  Selector : Selector  InputPortWidth=nbc*4  IndexOptions=Index vector (dialog)  Indices=[1: 4: nbc*4]  OutputSizes=1
  Selector1 : Selector  InputPortWidth=nbc*4  IndexOptions=Index vector (dialog)  Indices=[2: 4: nbc*4]  OutputSizes=1
  Selector2 : Selector  InputPortWidth=nbc*4  IndexOptions=Index vector (dialog)  Indices=[3: 4: nbc*4]  OutputSizes=1
  Selector3 : Selector  InputPortWidth=nbc*4  IndexOptions=Index vector (dialog)  Indices=[4: 4: nbc*4]  OutputSizes=1
  Simulink-PS Converter : nesl_utility/Simulink-PS Converter  PhysicalDomain=network_engine_domain  SubClassName=ps_input  LeftPortType=input  RightPortType=output  PseudoPeriodic=off  Frequencies=[]  NoiseDistribution=none  NoiseParameters=[]  Unit=1  AffineConversion=off  FilteringAndDerivatives=provide  SimscapeFilterOrder=1  InputFilterTimeConstant=0.001  UdotUserProvided=0
  Simulink-PS Converter1 : nesl_utility/Simulink-PS Converter  PhysicalDomain=network_engine_domain  SubClassName=ps_input  LeftPortType=input  RightPortType=output  PseudoPeriodic=off  Frequencies=[]  NoiseDistribution=none  NoiseParameters=[]  Unit=1  AffineConversion=off  FilteringAndDerivatives=provide  SimscapeFilterOrder=1  InputFilterTimeConstant=0.001  UdotUserProvided=0
  Unit Delay : UnitDelay  SampleTime=Ts  HasFrameUpgradeWarning=on
  Variable Resistor : fl_lib/Electrical/Electrical Elements/Variable Resistor  Rmin=1e-9 Ohm  thermalEnable=false  thermal_mass=1 J/K  i_specify=off  i_priority=None  i=0 A  i_nominal_specify=off  i_nominal_value=1  i_nominal_unit=A  v_specify=off  v_priority=None  v=0 V  v_nominal_specify=off  v_nominal_value=1  v_nominal_unit=V  T_specify=off  T_priority=None  T=300 K  T_nominal_specify=off  T_nominal_value=1  T_nominal_unit=K
  Voltage Sensor : fl_lib/Electrical/Electrical Sensors/Voltage Sensor
  +V : PMIOPort  Side=Right
  -V : PMIOPort  Port=2  Side=Right
  vi : Outport  VectorParamsAs1DForOutWhenUnconnected=off
  wires:
  S-Function/4 -> Bus Creator/2  "Idc(A)"
  Bus Creator/1 -> vi/1
  Vdc/1 -> S-Function/6
  [g1] -> S-Function/2
  [g2] -> S-Function/3
  [g3] -> S-Function/4
  [g4] -> S-Function/5
  Selector3/1 -> [g4]
  Selector2/1 -> [g3]
  Selector1/1 -> [g2]
  Selector/1 -> [g1]
  g/1 -> Selector/1, Selector1/1, Selector2/1, Selector3/1
  Saturation/1 -> Divide/1
  PS-Simulink Converter2/1 -> [Vnode_ssc]
  [Vnode_ssc] -> Unit Delay/1
  Divide/1 -> Simulink-PS Converter/1
  Unit Delay/1 -> S-Function/1  "Vbranch(V)"
  S-Function/1 -> Saturation/1
  S-Function/3 -> Bus Creator/1  "Vdc(V)"
  S-Function/2 -> Simulink-PS Converter1/1
  connections:
  PS-Simulink Converter2/LConn1 -- Voltage Sensor/RConn1
  Simulink-PS Converter/RConn1 -- Variable Resistor/LConn1
  Controlled Current Source/RConn1 -- Simulink-PS Converter1/RConn1
  Variable Resistor/LConn2 -- Voltage Sensor/RConn2 -- -V/RConn1 -- Controlled Current Source/RConn2
  Variable Resistor/RConn1 -- Voltage Sensor/LConn1 -- Controlled Current Source/LConn1 -- +V/RConn1

== system simetranss/Power converters/MATE_MMCarm ==
  note: note i is current going out from + terminal
  g : Inport
  blk : Inport  Port=2
  Bus Creator5 : BusCreator  Inputs=2
  C Function1 : CFunction  OutputCode=|  StartCode=state = initialValue;  InitializeConditionsCode=|  CodegenOutputCode=|  CodegenStartCode=state = initialValue;  CodegenInitializeConditionsCode=|  SampleTime=SampleTime  CustomCodeSettingLocation=ModelConfigurationParameters  initialValue=0  Ad=Ad  Bd2=Bd2  C=C  nbc=nbc  Z=Z  SampleTime=-1
      OutputCode=|
      | {
      | 
      | int ssx;
      | double Vcapasum, Ymmc, Zmmc, Vhist, Vterm;
      | double I;
      | 
      | Vcapasum=0;
      | I=(Vnodal- state_keep[0])* state_keep[1];  
      | 
      |     for (int k=0;k<nbc;k++){ //  % scan of cells to complete state-space iteration
      |         Vcap[k]=x_keep[k]+Bd2keep[k]*I;
      |         if (*(g_lower+k)<0.5) Vcapasum+=Vcap[k]; // sum all non-shorted capacitor voltages
      |     }
      | 
      | 
      |     Vhist=0;  // reset Vhist
      |     Zmmc=0;  // reset
      |     Vterm=  Vnodal;
      | 
      | 
      |     // we calculate the cells conduction states from the gate values.
      |     for (int k=0;k<nbc;k++){
      |         // ss=2-> lower IGBT/diode ON
      |         // ss=1-> upper IGBT/diode ON  //attention!!!!
      |         // ss=0-> hi-Z
      |         ssx=(int)gate[k];
      |         if (*(g_lower+k)>0.5) ssx=2;
      |         else if (*(g_upper+k)>0.5) ssx=1;
      |         else {
      |             if  (Vterm<0)  ssx=2;
      |             else if( Vterm>Vcapasum) ssx=1;
      |             else  ssx=0;
      |         }
      | 
      |         x_keep[k]=Ad[ssx]*Vcap[k];  //+Bd1[ssx]*I;    Bd1=0 avec backward Euler                                                          // note: with BE Bd1=0
      |         Vhist+=(C[ssx]*x_keep[k]);    //V_hist =V_hist + C(k)*state_tmp(k);  % compute Thevenin voltage
      | 
      |         Zmmc+=Z[ssx];  // Z = sum(C'.*Bd2 + D);  Y=inv(Z)
      | 
      |         Bd2keep[k]=Bd2[ssx];
      |         gate[k]=ssx;
      |         *(Vcap_out+k)=Vcap[k];
      |         }
      | 
      | 
      |     Ymmc=1/Zmmc;    // admittance= inverse of the sum of cell impedance
      |     Ihist=Vhist*Ymmc;  // history source
      | 
      |     state_keep[0]=Vhist;
      | 
      |     Y=Ymmc;
      | 
      |     state_keep[1]=Ymmc;
      | 
      |     Immc=0.0-I;
      | 
      | }
      InitializeConditionsCode=|
      | for (int i=0; i<nbc ;i++){
      |     x_keep[i]=0;
      |     Bd2keep[i]*0;
      |     Vc_state[i]=0;
      |     gate[i]=0;
      |     Vcap[i]=0;
      |     }
      |     
      |     state=0;
      |     state_keep[0]=0;
      |     state_keep[1]=0;
      CodegenOutputCode=|
      | {
      | 
      | int ssx;
      | double Vcapasum, Ymmc, Zmmc, Vhist, Vterm;
      | double I;
      | 
      | Vcapasum=0;
      | I=(Vnodal- state_keep[0])* state_keep[1];  
      | 
      |     for (int k=0;k<nbc;k++){ //  % scan of cells to complete state-space iteration
      |         Vcap[k]=x_keep[k]+Bd2keep[k]*I;
      |         if (*(g_lower+k)<0.5) Vcapasum+=Vcap[k]; // sum all non-shorted capacitor voltages
      |     }
      | 
      | 
      |     Vhist=0;  // reset Vhist
      |     Zmmc=0;  // reset
      |     Vterm=  Vnodal;
      | 
      | 
      |     // we calculate the cells conduction states from the gate values.
      |     for (int k=0;k<nbc;k++){
      |         // ss=2-> lower IGBT/diode ON
      |         // ss=1-> upper IGBT/diode ON  //attention!!!!
      |         // ss=0-> hi-Z
      |         ssx=(int)gate[k];
      |         if (*(g_lower+k)>0.5) ssx=2;
      |         else if (*(g_upper+k)>0.5) ssx=1;
      |         else {
      |             if  (Vterm<0)  ssx=2;
      |             else if( Vterm>Vcapasum) ssx=1;
      |             else  ssx=0;
      |         }
      | 
      |         x_keep[k]=Ad[ssx]*Vcap[k];  //+Bd1[ssx]*I;    Bd1=0 avec backward Euler                                                          // note: with BE Bd1=0
      |         Vhist+=(C[ssx]*x_keep[k]);    //V_hist =V_hist + C(k)*state_tmp(k);  % compute Thevenin voltage
      | 
      |         Zmmc+=Z[ssx];  // Z = sum(C'.*Bd2 + D);  Y=inv(Z)
      | 
      |         Bd2keep[k]=Bd2[ssx];
      |         gate[k]=ssx;
      |         *(Vcap_out+k)=Vcap[k];
      |         }
      | 
      | 
      |     Ymmc=1/Zmmc;    // admittance= inverse of the sum of cell impedance
      |     Ihist=Vhist*Ymmc;  // history source
      | 
      |     state_keep[0]=Vhist;
      | 
      |     Y=Ymmc;
      | 
      |     state_keep[1]=Ymmc;
      | 
      |     Immc=0.0-I;
      | 
      | }
      CodegenInitializeConditionsCode=|
      | for (int i=0; i<nbc ;i++){
      |     x_keep[i]=0;
      |     Bd2keep[i]*0;
      |     Vc_state[i]=0;
      |     gate[i]=0;
      |     Vcap[i]=0;
      |     }
      |     
      |     state=0;
      |     state_keep[0]=0;
      |     state_keep[1]=0;
  Controlled Current Source : fl_lib/Electrical/Electrical Sources/Controlled Current Source
  Divide : Product  Inputs=/
  PS-Simulink Converter2 : nesl_utility/PS-Simulink Converter  PhysicalDomain=network_engine_domain  SubClassName=ps_output  LeftPortType=input  RightPortType=output  PseudoPeriodic=off  Frequencies=[]  VectorFormat=inherit  Unit=inherit  AffineConversion=off
  Saturation : Saturate  UpperLimit=1e9  LowerLimit=0
  Simulink-PS Converter : nesl_utility/Simulink-PS Converter  PhysicalDomain=network_engine_domain  SubClassName=ps_input  LeftPortType=input  RightPortType=output  PseudoPeriodic=off  Frequencies=[]  NoiseDistribution=none  NoiseParameters=[]  Unit=1  AffineConversion=off  FilteringAndDerivatives=provide  SimscapeFilterOrder=1  InputFilterTimeConstant=0.001  UdotUserProvided=0
  Simulink-PS Converter1 : nesl_utility/Simulink-PS Converter  PhysicalDomain=network_engine_domain  SubClassName=ps_input  LeftPortType=input  RightPortType=output  PseudoPeriodic=off  Frequencies=[]  NoiseDistribution=none  NoiseParameters=[]  Unit=1  AffineConversion=off  FilteringAndDerivatives=provide  SimscapeFilterOrder=1  InputFilterTimeConstant=0.001  UdotUserProvided=0
  Subsystem : Subsystem  mask(MMC pulsing){nbc=nbc}
      mask prompts: nbc "Number of Cells"
      mask init:
      | igbtorder=[];
      | for i=1:nbc
      |     igbtorder=[igbtorder i i+nbc];
      | end
      | igbtorder;
  Unit Delay : UnitDelay  SampleTime=Ts  HasFrameUpgradeWarning=on
  Variable Resistor : fl_lib/Electrical/Electrical Elements/Variable Resistor  Rmin=1e-8 Ohm  thermalEnable=false  thermal_mass=1 J/K  i_specify=off  i_priority=None  i=0 A  i_nominal_specify=off  i_nominal_value=1  i_nominal_unit=A  v_specify=off  v_priority=None  v=0 V  v_nominal_specify=off  v_nominal_value=1  v_nominal_unit=V  T_specify=off  T_priority=None  T=300 K  T_nominal_specify=off  T_nominal_value=1  T_nominal_unit=K
  Voltage Sensor : fl_lib/Electrical/Electrical Sensors/Voltage Sensor
  +V : PMIOPort  Side=Left
  -V : PMIOPort  Port=2  Side=Left
  iv : Outport  VectorParamsAs1DForOutWhenUnconnected=off
  Vc : Outport  Port=2  VectorParamsAs1DForOutWhenUnconnected=off
  wires:
  Saturation/1 -> Divide/1
  Divide/1 -> Simulink-PS Converter/1
  C Function1/2 -> Simulink-PS Converter1/1
  [Vnode_ssc] -> Unit Delay/1
  PS-Simulink Converter2/1 -> [Vnode_ssc]
  blk/1 -> Subsystem/2(en)
  Subsystem/2(outN) -> C Function1/2
  g/1 -> Subsystem/1(gup)
  Subsystem/1(out) -> C Function1/1
  Bus Creator5/1 -> iv/1
  Unit Delay/1 -> C Function1/3, Bus Creator5/2  "Vc"
  C Function1/1 -> Saturation/1
  C Function1/3 -> Vc/1
  C Function1/4 -> Bus Creator5/1  "Iin"
  connections:
  Controlled Current Source/RConn1 -- Simulink-PS Converter1/RConn1
  PS-Simulink Converter2/LConn1 -- Voltage Sensor/RConn1
  Variable Resistor/RConn1 -- +V/RConn1 -- Controlled Current Source/LConn1 -- Voltage Sensor/LConn1
  Variable Resistor/LConn2 -- -V/RConn1 -- Controlled Current Source/RConn2 -- Voltage Sensor/RConn2
  Simulink-PS Converter/RConn1 -- Variable Resistor/LConn1

== system simetranss/Power converters/Oversampled Switching function 2-level IGBT//diode inverter (3ph) ==
  g : Inport
  Demux5 : Demux  Outputs=[2 2 2]
  Phase Splitter : ee_lib/Connectors & References/Phase Splitter
  Switching Function Interpolating 2-level inverter : $bdroot/Power converters/Switching Function  Interpolating 2-level inverter  Ron=Ron  Gp=Rsnubber  Gi=Csnubber  Ts=Ts  dc_short_resistance=0.1
  Switching Function Interpolating 2-level inverter1 : $bdroot/Power converters/Switching Function  Interpolating 2-level inverter  Ron=Ron  Gp=Rsnubber  Gi=Csnubber  Ts=Ts  dc_short_resistance=0.1
  Switching Function Interpolating 2-level inverter2 : $bdroot/Power converters/Switching Function  Interpolating 2-level inverter  Ron=Ron  Gp=Rsnubber  Gi=Csnubber  Ts=Ts  dc_short_resistance=0.1
  V+ : PMIOPort  Side=Left
  abc : PMIOPort  Port=2  Side=Right
  V- : PMIOPort  Port=3  Side=Left
  wires:
  Demux5/1 -> Switching Function Interpolating 2-level inverter/1
  Demux5/2 -> Switching Function Interpolating 2-level inverter1/1
  g/1 -> Demux5/1
  Demux5/3 -> Switching Function Interpolating 2-level inverter2/1
  connections:
  Switching Function Interpolating 2-level inverter2/LConn1 -- Phase Splitter/RConn3
  Switching Function Interpolating 2-level inverter1/LConn1 -- Phase Splitter/RConn2
  Switching Function Interpolating 2-level inverter/LConn1 -- Phase Splitter/RConn1
  abc/RConn1 -- Phase Splitter/LConn1
  Switching Function Interpolating 2-level inverter2/RConn1 -- V+/RConn1 -- Switching Function Interpolating 2-level inverter/RConn1 -- Switching Function Interpolating 2-level inverter1/RConn1
  Switching Function Interpolating 2-level inverter2/RConn2 -- V-/RConn1 -- Switching Function Interpolating 2-level inverter/RConn2 -- Switching Function Interpolating 2-level inverter1/RConn2
